simulink model "Quadcopter"  (R2023a)
settings: Solver=FixedStepAuto  StartTime=0.0  StopTime=500  FixedStep=step_size  RelTol=1e-3
undefined symbols (not defined in the file or in its folder): gain, init
settings Model: Creator=Sebastian  LastModifiedBy=juanv
settings OptimizationCC: ReuseModelBlockBuffer=off

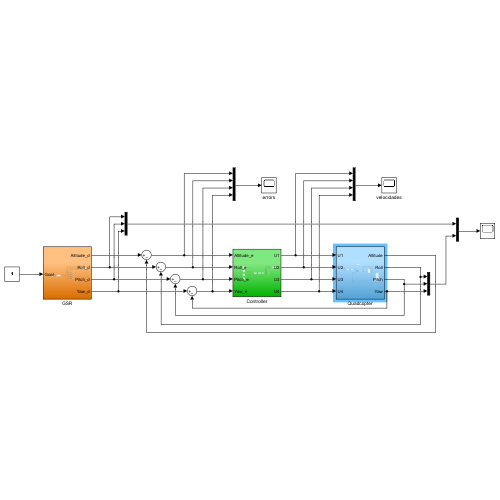
[thumbnail: Simulink's stored preview of the top-level diagram]
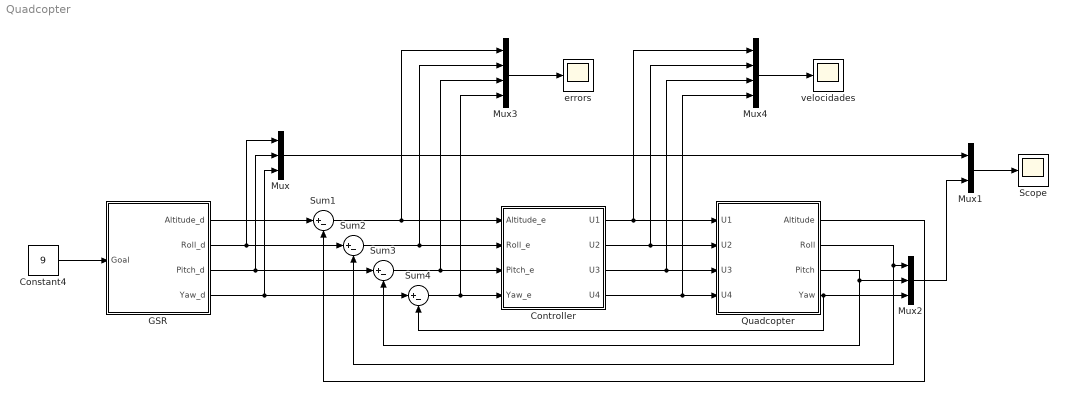
== system Quadcopter ==
  Constant4 : Constant  Value=9
  Controller : Subsystem
  GSR : Subsystem
  Mux : Mux  Inputs=3
  Mux1 : Mux  Inputs=2
  Mux2 : Mux  Inputs=3
  Mux3 : Mux
  Mux4 : Mux
  Quadcopter : Subsystem
  Scope : Scope
  Sum{1..4} (4 alike) : Sum  Inputs=|+-
  errors : Scope
  velocidades : Scope
  wires:
  Constant4/1 -> GSR/1(Goal)
  GSR/2(Roll_d) -> Mux/1, Sum2/1
  Quadcopter/2(Roll) -> Sum2/2, Mux2/1
  GSR/3(Pitch_d) -> Mux/2, Sum3/1
  GSR/4(Yaw_d) -> Mux/3, Sum4/1
  Quadcopter/3(Pitch) -> Sum3/2, Mux2/2
  Quadcopter/4(Yaw) -> Mux2/3, Sum4/2
  Sum2/1 -> Mux3/2, Controller/2(Roll_e)
  Sum3/1 -> Mux3/3, Controller/3(Pitch_e)
  Sum4/1 -> Controller/4(Yaw_e), Mux3/4
  Mux/1 -> Mux1/1
  Mux2/1 -> Mux1/2
  Mux1/1 -> Scope/1
  Quadcopter/1(Altitude) -> Sum1/2
  GSR/1(Altitude_d) -> Sum1/1
  Sum1/1 -> Mux3/1, Controller/1(Altitude_e)
  Controller/1(U1) -> Mux4/1, Quadcopter/1(U1)
  Controller/2(U2) -> Mux4/2, Quadcopter/2(U2)
  Controller/3(U3) -> Mux4/3, Quadcopter/3(U3)
  Controller/4(U4) -> Mux4/4, Quadcopter/4(U4)
  Mux3/1 -> errors/1
  Mux4/1 -> velocidades/1

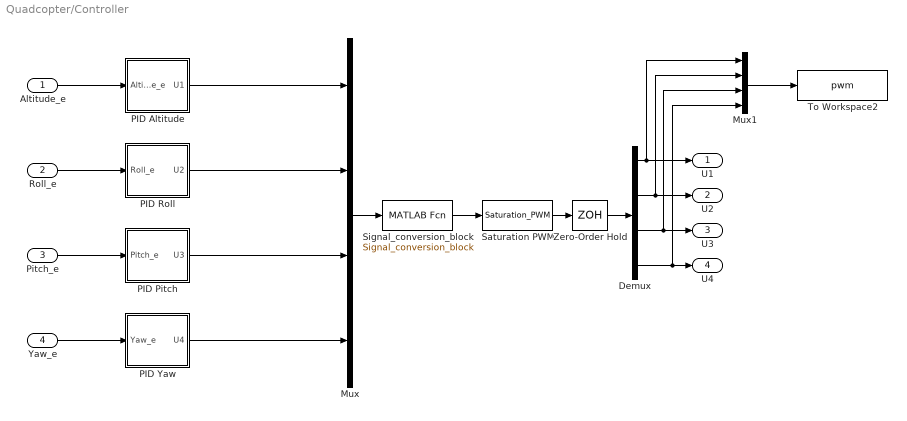
== system Quadcopter/Controller ==
  Altitude_e : Inport
  Roll_e : Inport  Port=2
  Pitch_e : Inport  Port=3
  Yaw_e : Inport  Port=4
  Demux : Demux
  Mux : Mux
  Mux1 : Mux
  PID Altitude : Subsystem
  PID Pitch : Subsystem
  PID Roll : Subsystem
  PID Yaw : Subsystem
  Saturation PWM : MATLABFcn  MATLABFcn=Saturation_PWM  OutputDimensions=4
  Signal_conversion_block : MATLABFcn  MATLABFcn=Signal_conversion_block  OutputDimensions=4
  To Workspace2 : ToWorkspace  VariableName=pwm  SampleTime=-1
  Zero-Order Hold : ZeroOrderHold  SampleTime=-1
  U1 : Outport
  U2 : Outport  Port=2
  U3 : Outport  Port=3
  U4 : Outport  Port=4
  wires:
  Mux/1 -> Signal_conversion_block/1
  Signal_conversion_block/1 -> Saturation PWM/1
  Demux/1 -> Mux1/1, U1/1
  Demux/3 -> Mux1/3, U3/1
  Roll_e/1 -> PID Roll/1(Roll_e)
  Demux/2 -> Mux1/2, U2/1
  Demux/4 -> Mux1/4, U4/1
  Yaw_e/1 -> PID Yaw/1(Yaw_e)
  PID Yaw/1(U4) -> Mux/4
  Pitch_e/1 -> PID Pitch/1(Pitch_e)
  PID Pitch/1(U3) -> Mux/3
  PID Roll/1(U2) -> Mux/2
  Altitude_e/1 -> PID Altitude/1(Altitude_e)
  PID Altitude/1(U1) -> Mux/1
  Mux1/1 -> To Workspace2/1
  Saturation PWM/1 -> Zero-Order Hold/1
  Zero-Order Hold/1 -> Demux/1

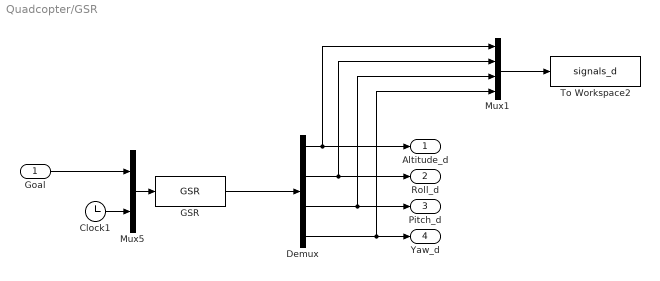
== system Quadcopter/GSR ==
  Goal : Inport
  Clock1 : Clock
  Demux : Demux
  GSR : MATLABFcn  MATLABFcn=GSR  OutputDimensions=4
  Mux1 : Mux
  Mux5 : Mux  Inputs=2
  To Workspace2 : ToWorkspace  VariableName=signals_d  SampleTime=-1
  Altitude_d : Outport
  Roll_d : Outport  Port=2
  Pitch_d : Outport  Port=3
  Yaw_d : Outport  Port=4
  wires:
  Demux/1 -> Mux1/1, Altitude_d/1
  Demux/4 -> Mux1/4, Yaw_d/1
  Mux5/1 -> GSR/1
  Goal/1 -> Mux5/1
  Demux/2 -> Mux1/2, Roll_d/1
  Clock1/1 -> Mux5/2
  Demux/3 -> Mux1/3, Pitch_d/1
  Mux1/1 -> To Workspace2/1
  GSR/1 -> Demux/1

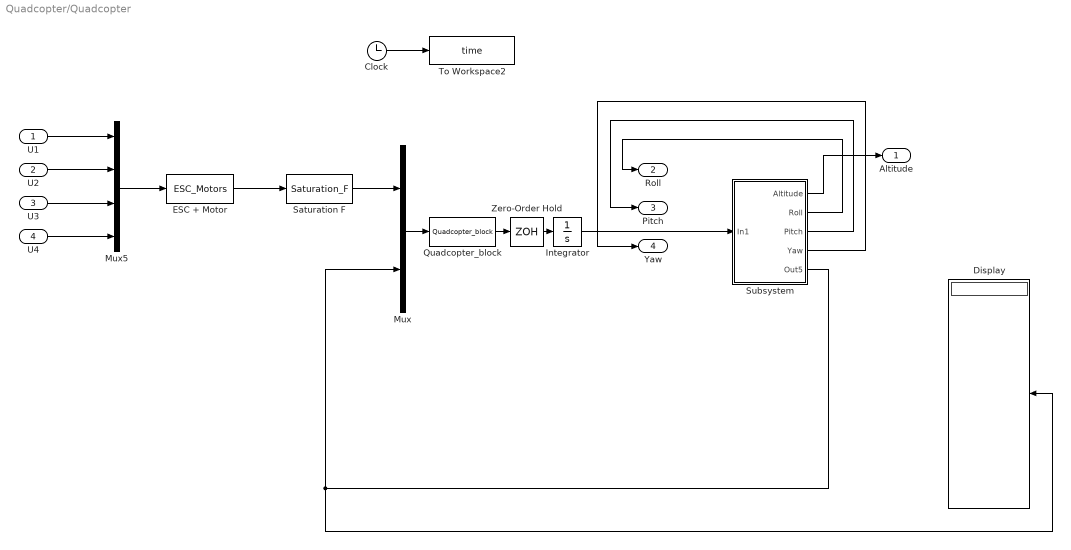
== system Quadcopter/Quadcopter ==
  U1 : Inport
  U2 : Inport  Port=2
  U3 : Inport  Port=3
  U4 : Inport  Port=4
  Clock : Clock
  Display : Display
  ESC + Motor : MATLABFcn  MATLABFcn=ESC_Motors  OutputDimensions=4
  Integrator : Integrator  InitialCondition=[init.dx init.dy init.dz init.phi init.theta init.psi init.p init.q init.r]
  Mux : Mux  Inputs=2
  Mux5 : Mux
  Quadcopter_block : MATLABFcn  MATLABFcn=Quadcopter_block  OutputDimensions=9
  Saturation F : MATLABFcn  MATLABFcn=Saturation_F  OutputDimensions=4
  Subsystem : Subsystem
  To Workspace2 : ToWorkspace  VariableName=time  SampleTime=-1
  Zero-Order Hold : ZeroOrderHold  SampleTime=-1
  Altitude : Outport
  Roll : Outport  Port=2
  Pitch : Outport  Port=3
  Yaw : Outport  Port=4
  wires:
  Mux/1 -> Quadcopter_block/1
  Clock/1 -> To Workspace2/1
  U1/1 -> Mux5/1
  U4/1 -> Mux5/4
  Saturation F/1 -> Mux/1
  U2/1 -> Mux5/2
  U3/1 -> Mux5/3
  ESC + Motor/1 -> Saturation F/1
  Mux5/1 -> ESC + Motor/1
  Quadcopter_block/1 -> Zero-Order Hold/1
  Zero-Order Hold/1 -> Integrator/1
  Subsystem/5(Out5) -> Mux/2, Display/1
  Integrator/1 -> Subsystem/1(In1)
  Subsystem/1(Altitude) -> Altitude/1
  Subsystem/2(Roll) -> Roll/1
  Subsystem/3(Pitch) -> Pitch/1
  Subsystem/4(Yaw) -> Yaw/1

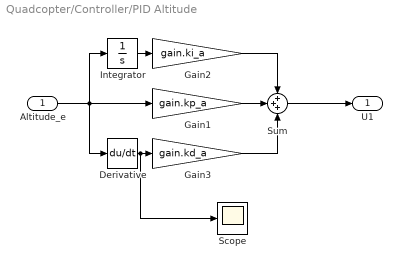
== system Quadcopter/Controller/PID Altitude ==
  Altitude_e : Inport
  Derivative : Derivative
  Gain1 : Gain  Gain=gain.kp_a
  Gain2 : Gain  Gain=gain.ki_a
  Gain3 : Gain  Gain=gain.kd_a
  Integrator : Integrator
  Scope : Scope
  Sum : Sum  Inputs=+++
  U1 : Outport
  wires:
  Gain1/1 -> Sum/2
  Sum/1 -> U1/1
  Derivative/1 -> Scope/1, Gain3/1
  Integrator/1 -> Gain2/1
  Gain3/1 -> Sum/3
  Gain2/1 -> Sum/1
  Altitude_e/1 -> Gain1/1, Integrator/1, Derivative/1

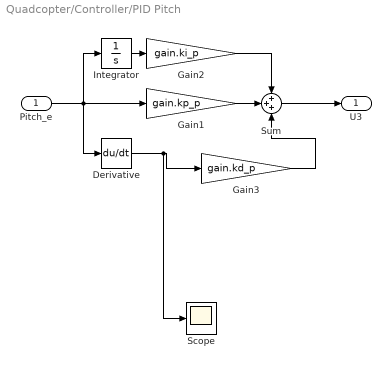
== system Quadcopter/Controller/PID Pitch ==
  Pitch_e : Inport
  Derivative : Derivative
  Gain1 : Gain  Gain=gain.kp_p
  Gain2 : Gain  Gain=gain.ki_p
  Gain3 : Gain  Gain=gain.kd_p
  Integrator : Integrator
  Scope : Scope
  Sum : Sum  Inputs=+++
  U3 : Outport
  wires:
  Pitch_e/1 -> Derivative/1, Integrator/1, Gain1/1
  Gain1/1 -> Sum/2
  Derivative/1 -> Scope/1, Gain3/1
  Sum/1 -> U3/1
  Integrator/1 -> Gain2/1
  Gain3/1 -> Sum/3
  Gain2/1 -> Sum/1

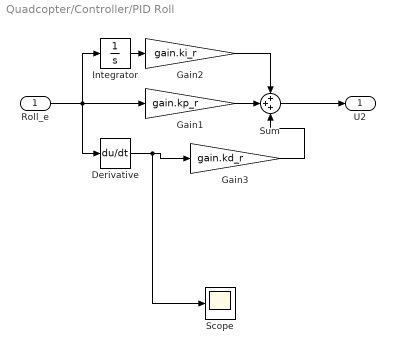
== system Quadcopter/Controller/PID Roll ==
  Roll_e : Inport
  Derivative : Derivative
  Gain1 : Gain  Gain=gain.kp_r
  Gain2 : Gain  Gain=gain.ki_r
  Gain3 : Gain  Gain=gain.kd_r
  Integrator : Integrator
  Scope : Scope
  Sum : Sum  Inputs=+++
  U2 : Outport
  wires:
  Roll_e/1 -> Derivative/1, Integrator/1, Gain1/1
  Gain2/1 -> Sum/1
  Gain3/1 -> Sum/3
  Integrator/1 -> Gain2/1
  Derivative/1 -> Scope/1, Gain3/1
  Sum/1 -> U2/1
  Gain1/1 -> Sum/2

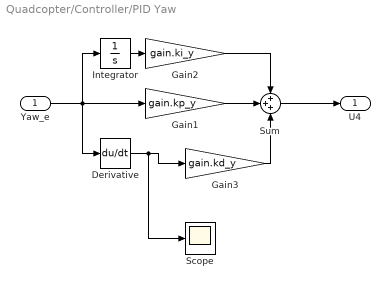
== system Quadcopter/Controller/PID Yaw ==
  Yaw_e : Inport
  Derivative : Derivative
  Gain1 : Gain  Gain=gain.kp_y
  Gain2 : Gain  Gain=gain.ki_y
  Gain3 : Gain  Gain=gain.kd_y
  Integrator : Integrator
  Scope : Scope
  Sum : Sum  Inputs=+++
  U4 : Outport
  wires:
  Yaw_e/1 -> Derivative/1, Integrator/1, Gain1/1
  Gain1/1 -> Sum/2
  Derivative/1 -> Scope/1, Gain3/1
  Sum/1 -> U4/1
  Integrator/1 -> Gain2/1
  Gain3/1 -> Sum/3
  Gain2/1 -> Sum/1

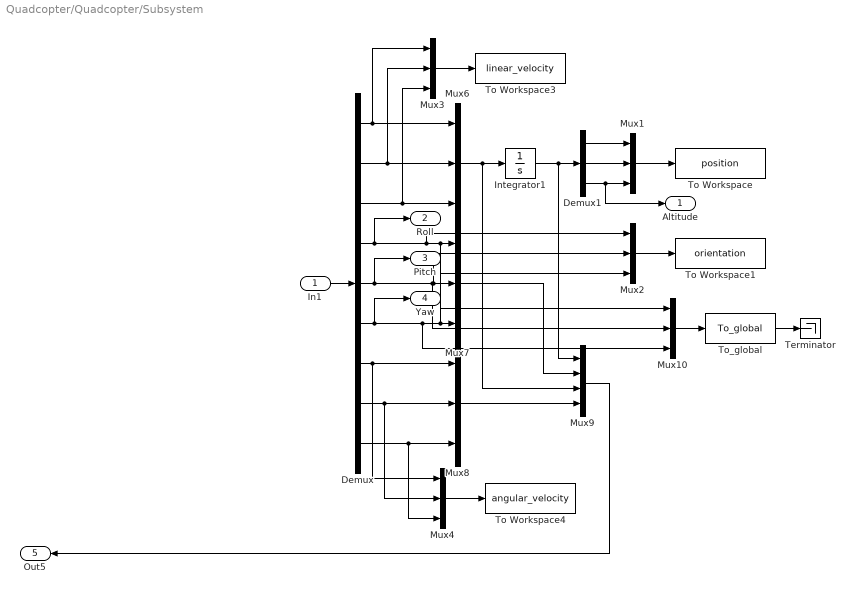
== system Quadcopter/Quadcopter/Subsystem ==
  In1 : Inport
  Demux : Demux  Outputs=9
  Demux1 : Demux  Outputs=3
  Integrator1 : Integrator  InitialCondition=[init.x init.y init.z]
  Mux{1..4,6..8,10} (8 alike) : Mux  Inputs=3
  Mux9 : Mux
  Terminator : Terminator
  To Workspace : ToWorkspace  VariableName=position  SampleTime=-1
  To Workspace1 : ToWorkspace  VariableName=orientation  SampleTime=-1
  To Workspace3 : ToWorkspace  VariableName=linear_velocity  SampleTime=-1
  To Workspace4 : ToWorkspace  VariableName=angular_velocity  SampleTime=-1
  To_global : MATLABFcn  MATLABFcn=To_global  OutputDimensions=1
  Altitude : Outport
  Roll : Outport  Port=2
  Pitch : Outport  Port=3
  Yaw : Outport  Port=4
  Out5 : Outport  Port=5
  wires:
  Demux/4 -> Roll/1, Mux10/1, Mux7/1, Mux2/1
  Mux10/1 -> To_global/1
  Demux/3 -> Mux6/3, Mux3/3
  Demux1/3 -> Altitude/1, Mux1/3
  Mux2/1 -> To Workspace1/1
  Mux4/1 -> To Workspace4/1
  In1/1 -> Demux/1
  Integrator1/1 -> Mux9/1, Demux1/1
  Demux/9 -> Mux4/3, Mux8/3
  Demux/5 -> Pitch/1, Mux10/2, Mux7/2, Mux2/2
  Demux1/1 -> Mux1/1
  Demux/7 -> Mux4/1, Mux8/1
  Demux/6 -> Yaw/1, Mux10/3, Mux7/3, Mux2/3
  Demux/2 -> Mux3/2, Mux6/2
  Demux/1 -> Mux6/1, Mux3/1
  Mux1/1 -> To Workspace/1
  To_global/1 -> Terminator/1
  Mux3/1 -> To Workspace3/1
  Demux/8 -> Mux4/2, Mux8/2
  Demux1/2 -> Mux1/2
  Mux7/1 -> Mux9/2
  Mux6/1 -> Mux9/3, Integrator1/1
  Mux8/1 -> Mux9/4
  Mux9/1 -> Out5/1
